simulink model "HopperPlant_optimisation"  (R2024b)
settings: Solver=VariableStepAuto  StartTime=0.0  StopTime=60  RelTol=1e-3
values from neighbouring files (symbols this model uses):
  height_setpoint = 20    [Visualisation.m]    (also in optimisation.m)
  Kd_z = 50.7347    [Visualisation.m]    (also in optimisation.m)
  Ki_z = 0.35426    [Visualisation.m]    (also in optimisation.m)
  Kp_z = 90.3674    [Visualisation.m]    (also in optimisation.m)
  max_thrust = 20    [Visualisation.m]    (also in optimisation.m)
  x_setpoint = 2    [Visualisation.m]    (also in optimisation.m)
  y_setpoint = 2    [Visualisation.m]    (also in optimisation.m)
undefined symbols (not defined in the file or in its folder): DiscIntNeverNeededParam, Kd_alpha, Kd_beta, Kd_x, Kd_y, Ki_alpha, Ki_beta, Ki_x, Ki_y, Kp_alpha, Kp_beta, Kp_x, Kp_y
libraries: slpidlib x15
(part 2 of 2)

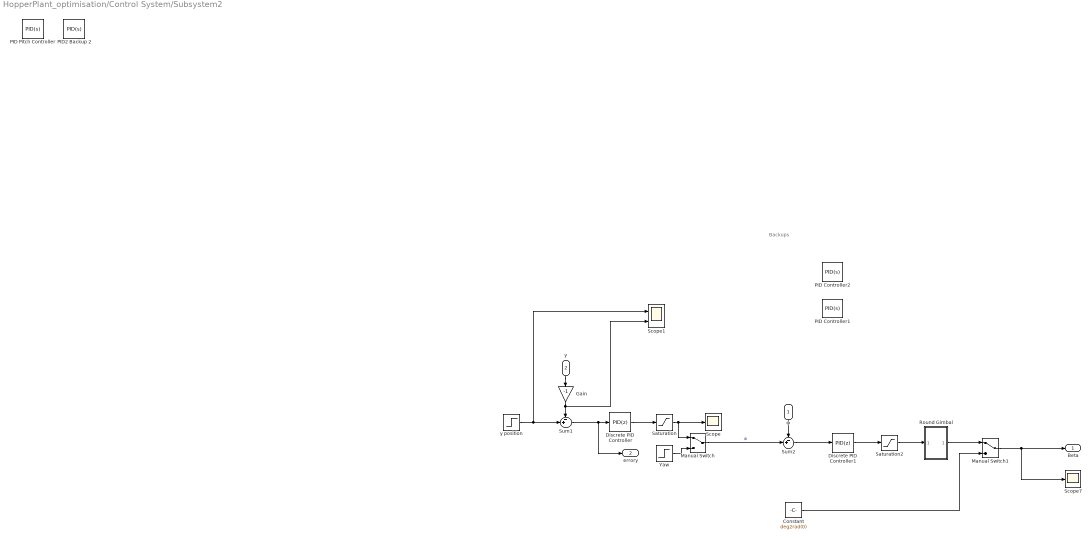
== system HopperPlant_optimisation/Control System/Subsystem2 ==
  note: Backups
  Φ : Inport
  y : Inport  Port=2
  Constant : Constant  Value=deg2rad(0)  SampleTime=0.01
  Discrete PID Controller : slpidlib/PID Controller  Controller=PID  Form=Parallel  TimeDomain=Discrete-time  UseExternalTs=off  SampleTime=-1  IntegratorMethod=Forward Euler  FilterMethod=Forward Euler  ControllerParametersSource=internal  P=Kp_y  I=Ki_y  UseKiTs=off  D=Kd_y  UseExternalDerivativeSource=off  N=100  UseFilter=off  TunerSelectOption=Transfer Function Based (PID Tuner App)  InitialConditionSource=internal  InitialConditionForIntegrator=0  InitialConditionForFilter=0  DifferentiatorICPrevScaledInput=0  ExternalReset=none  TrackingMode=off  Kt=1  LimitOutput=off  SatLimitsSource=internal  UpperSaturationLimit=inf  LowerSaturationLimit=-inf  LinearizeAsGain=off  AntiWindupMode=none  Kb=1  LimitIntegrator=off  UpperIntegratorSaturationLimit=inf  LowerIntegratorSaturationLimit=-inf  POutMin=[]  POutMax=[]  IOutMin=[]  IOutMax=[]  DOutMin=[]  DOutMax=[]  NOutMin=[]  NOutMax=[]  SumOutMin=[]  SumOutMax=[]  SaturationOutMin=[]  SaturationOutMax=[]  PParamMin=[]  PParamMax=[]  IParamMin=[]  IParamMax=[]  DParamMin=[]  DParamMax=[]  NParamMin=[]  NParamMax=[]  KbParamMin=[]  KbParamMax=[]  KtParamMin=[]  KtParamMax=[]  KbOutMin=[]  KbOutMax=[]  KtOutMin=[]  KtOutMax=[]  IntegratorOutMin=[]  IntegratorOutMax=[]  FilterOutMin=[]  FilterOutMax=[]  SumI1OutMin=[]  SumI1OutMax=[]  SumI2OutMin=[]  SumI2OutMax=[]  SumI3OutMin=[]  SumI3OutMax=[]  SumI4OutMin=[]  SumI4OutMax=[]  SumDOutMin=[]  SumDOutMax=[]  DifferentiatorOutMin=[]  DifferentiatorOutMax=[]  FilterDiffOutCoefMin=[]  FilterDiffOutCoefMax=[]  ReciprocalOutMin=[]  ReciprocalOutMax=[]  SumDenOutMin=[]  SumDenOutMax=[]  SumNumOutMin=[]  SumNumOutMax=[]  DivideOutMin=[]  DivideOutMax=[]  UdiffTsProdOutMin=[]  UdiffTsProdOutMax=[]  NTsProdOutMin=[]  NTsProdOutMax=[]  UintegralTsProdOutMin=[]  UintegralTsProdOutMax=[]  UngainTsProdOutMin=[]  UngainTsProdOutMax=[]  ClampingZeroOutDataTypeStr=Inherit: Inherit via back propagation  ClampingZeroOutMin=[]  ClampingZeroOutMax=[]  FilterDenConstantOutDataTypeStr=Inherit: Inherit via back propagation  FilterDenConstantOutMin=[]  FilterDenConstantOutMax=[]  PCopyOutDataTypeStr=Inherit: Inherit via back propagation  PCopyOutMin=[]  PCopyOutMax=[]  NCopyOutDataTypeStr=Inherit: Inherit via back propagation  NCopyOutMin=[]  NCopyOutMax=[]  IntegratorContinuousStateAttributes=''  IntegratorStateMustResolveToSignalObject=off  IntegratorRTWStateStorageClass=Auto  FilterContinuousStateAttributes=''  FilterStateMustResolveToSignalObject=off  FilterRTWStateStorageClass=Auto  ParallelPVariant=InternalParameters  IdealPVariant=Disabled  IVariant=InternalParameters  DVariant=InternalParameters  IntegratorVariant=Discrete  SatVariant=Disabled  AWVariant=Passthrough  PCopyVariant=Disabled  TRVariant=Disabled  FdbkBlocksVariant=Forward  IdealPFdbkVariant=Disabled  SatFdbkVariant=Disabled  DerivativeFilterVariant=Differentiator  NVariant=Passthrough  NCopyVariant=Disabled_SignalSpec  FilterICVariant=InternalICsDifferentiator  IntegratorICVariant=InternalICs  ExternalResetVariant=Disabled  TRSumVariant=Passthrough  SumFdbkVariant=Disabled  SumVariant=Sum_PID  TsampFilterVariant=InternalTs  TsampNgainVariant=Passthrough  TsampIntegralVariant=Disabled_SignalSpec  ExternalSaturationOutDataTypeStr=Inherit: Same as second input  DerivativeSourceVariant=ErrorSignal  PreIntVariant=InternalPreInt
      settings: LibrarySourceBlock=simulink/Discrete/Discrete PID Controller
  Discrete PID Controller1 : slpidlib/PID Controller  Controller=PID  Form=Parallel  TimeDomain=Discrete-time  UseExternalTs=off  SampleTime=-1  IntegratorMethod=Forward Euler  FilterMethod=Forward Euler  ControllerParametersSource=internal  P=Kp_beta  I=Ki_beta  UseKiTs=off  D=Kd_beta  UseExternalDerivativeSource=off  N=100  UseFilter=on  TunerSelectOption=Transfer Function Based (PID Tuner App)  InitialConditionSource=internal  InitialConditionForIntegrator=0  InitialConditionForFilter=0  DifferentiatorICPrevScaledInput=0  ExternalReset=none  TrackingMode=off  Kt=1  LimitOutput=off  SatLimitsSource=internal  UpperSaturationLimit=inf  LowerSaturationLimit=-inf  LinearizeAsGain=off  AntiWindupMode=none  Kb=1  LimitIntegrator=off  UpperIntegratorSaturationLimit=inf  LowerIntegratorSaturationLimit=-inf  POutMin=[]  POutMax=[]  IOutMin=[]  IOutMax=[]  DOutMin=[]  DOutMax=[]  NOutMin=[]  NOutMax=[]  SumOutMin=[]  SumOutMax=[]  SaturationOutMin=[]  SaturationOutMax=[]  PParamMin=[]  PParamMax=[]  IParamMin=[]  IParamMax=[]  DParamMin=[]  DParamMax=[]  NParamMin=[]  NParamMax=[]  KbParamMin=[]  KbParamMax=[]  KtParamMin=[]  KtParamMax=[]  KbOutMin=[]  KbOutMax=[]  KtOutMin=[]  KtOutMax=[]  IntegratorOutMin=[]  IntegratorOutMax=[]  FilterOutMin=[]  FilterOutMax=[]  SumI1OutMin=[]  SumI1OutMax=[]  SumI2OutMin=[]  SumI2OutMax=[]  SumI3OutMin=[]  SumI3OutMax=[]  SumI4OutMin=[]  SumI4OutMax=[]  SumDOutMin=[]  SumDOutMax=[]  DifferentiatorOutMin=[]  DifferentiatorOutMax=[]  FilterDiffOutCoefMin=[]  FilterDiffOutCoefMax=[]  ReciprocalOutMin=[]  ReciprocalOutMax=[]  SumDenOutMin=[]  SumDenOutMax=[]  SumNumOutMin=[]  SumNumOutMax=[]  DivideOutMin=[]  DivideOutMax=[]  UdiffTsProdOutMin=[]  UdiffTsProdOutMax=[]  NTsProdOutMin=[]  NTsProdOutMax=[]  UintegralTsProdOutMin=[]  UintegralTsProdOutMax=[]  UngainTsProdOutMin=[]  UngainTsProdOutMax=[]  ClampingZeroOutDataTypeStr=Inherit: Inherit via back propagation  ClampingZeroOutMin=[]  ClampingZeroOutMax=[]  FilterDenConstantOutDataTypeStr=Inherit: Inherit via back propagation  FilterDenConstantOutMin=[]  FilterDenConstantOutMax=[]  PCopyOutDataTypeStr=Inherit: Inherit via back propagation  PCopyOutMin=[]  PCopyOutMax=[]  NCopyOutDataTypeStr=Inherit: Inherit via back propagation  NCopyOutMin=[]  NCopyOutMax=[]  IntegratorContinuousStateAttributes=''  IntegratorStateMustResolveToSignalObject=off  IntegratorRTWStateStorageClass=Auto  FilterContinuousStateAttributes=''  FilterStateMustResolveToSignalObject=off  FilterRTWStateStorageClass=Auto  ParallelPVariant=InternalParameters  IdealPVariant=Disabled  IVariant=InternalParameters  DVariant=InternalParameters  IntegratorVariant=Discrete  SatVariant=Disabled  AWVariant=Passthrough  PCopyVariant=Disabled  TRVariant=Disabled  FdbkBlocksVariant=Forward  IdealPFdbkVariant=Disabled  SatFdbkVariant=Disabled  DerivativeFilterVariant=ForwardEulerFilter  NVariant=InternalParameters  NCopyVariant=Disabled  FilterICVariant=InternalICsFilter  IntegratorICVariant=InternalICs  ExternalResetVariant=Disabled  TRSumVariant=Passthrough  SumFdbkVariant=Disabled  SumVariant=Sum_PID  TsampFilterVariant=InternalTs  TsampNgainVariant=Passthrough  TsampIntegralVariant=Disabled_SignalSpec  ExternalSaturationOutDataTypeStr=Inherit: Same as second input  DerivativeSourceVariant=ErrorSignal  PreIntVariant=InternalPreInt
      settings: LibrarySourceBlock=hdlsllib/Discrete/Discrete PID Controller
  Gain : Gain  Gain=-1
  Manual Switch : ManualSwitch
  Manual Switch1 : ManualSwitch
  PID Controller1 : slpidlib/PID Controller  Controller=PID  Form=Parallel  TimeDomain=Continuous-time  UseExternalTs=off  SampleTime=-1  IntegratorMethod=Forward Euler  FilterMethod=Forward Euler  ControllerParametersSource=internal  P=0.001  I=0  UseKiTs=off  D=0.00250  UseExternalDerivativeSource=off  N=100  UseFilter=on  TunerSelectOption=Transfer Function Based (PID Tuner App)  InitialConditionSource=internal  InitialConditionForIntegrator=0  InitialConditionForFilter=0  DifferentiatorICPrevScaledInput=0  ExternalReset=none  TrackingMode=off  Kt=1  LimitOutput=off  SatLimitsSource=internal  UpperSaturationLimit=inf  LowerSaturationLimit=-inf  LinearizeAsGain=on  AntiWindupMode=none  Kb=1  LimitIntegrator=off  UpperIntegratorSaturationLimit=inf  LowerIntegratorSaturationLimit=-inf  POutMin=[]  POutMax=[]  IOutMin=[]  IOutMax=[]  DOutMin=[]  DOutMax=[]  NOutMin=[]  NOutMax=[]  SumOutMin=[]  SumOutMax=[]  SaturationOutMin=[]  SaturationOutMax=[]  PParamMin=[]  PParamMax=[]  IParamMin=[]  IParamMax=[]  DParamMin=[]  DParamMax=[]  NParamMin=[]  NParamMax=[]  KbParamMin=[]  KbParamMax=[]  KtParamMin=[]  KtParamMax=[]  KbOutMin=[]  KbOutMax=[]  KtOutMin=[]  KtOutMax=[]  IntegratorOutMin=[]  IntegratorOutMax=[]  FilterOutMin=[]  FilterOutMax=[]  SumI1OutMin=[]  SumI1OutMax=[]  SumI2OutMin=[]  SumI2OutMax=[]  SumI3OutMin=[]  SumI3OutMax=[]  SumI4OutMin=[]  SumI4OutMax=[]  SumDOutMin=[]  SumDOutMax=[]  DifferentiatorOutMin=[]  DifferentiatorOutMax=[]  FilterDiffOutCoefMin=[]  FilterDiffOutCoefMax=[]  ReciprocalOutMin=[]  ReciprocalOutMax=[]  SumDenOutMin=[]  SumDenOutMax=[]  SumNumOutMin=[]  SumNumOutMax=[]  DivideOutMin=[]  DivideOutMax=[]  UdiffTsProdOutMin=[]  UdiffTsProdOutMax=[]  NTsProdOutMin=[]  NTsProdOutMax=[]  UintegralTsProdOutMin=[]  UintegralTsProdOutMax=[]  UngainTsProdOutMin=[]  UngainTsProdOutMax=[]  ClampingZeroOutDataTypeStr=Inherit: Inherit via back propagation  ClampingZeroOutMin=[]  ClampingZeroOutMax=[]  FilterDenConstantOutDataTypeStr=Inherit: Inherit via back propagation  FilterDenConstantOutMin=[]  FilterDenConstantOutMax=[]  PCopyOutDataTypeStr=Inherit: Inherit via back propagation  PCopyOutMin=[]  PCopyOutMax=[]  NCopyOutDataTypeStr=Inherit: Inherit via back propagation  NCopyOutMin=[]  NCopyOutMax=[]  IntegratorContinuousStateAttributes=''  IntegratorStateMustResolveToSignalObject=off  IntegratorRTWStateStorageClass=Auto  FilterContinuousStateAttributes=''  FilterStateMustResolveToSignalObject=off  FilterRTWStateStorageClass=Auto  ParallelPVariant=InternalParameters  IdealPVariant=Disabled  IVariant=InternalParameters  DVariant=InternalParameters  IntegratorVariant=Continuous  SatVariant=Disabled  AWVariant=Passthrough  PCopyVariant=Disabled  TRVariant=Disabled  FdbkBlocksVariant=Forward  IdealPFdbkVariant=Disabled  SatFdbkVariant=Disabled  DerivativeFilterVariant=ContFilter  NVariant=InternalParameters  NCopyVariant=Disabled  FilterICVariant=InternalICsFilter  IntegratorICVariant=InternalICs  ExternalResetVariant=Disabled  TRSumVariant=Passthrough  SumFdbkVariant=Disabled  SumVariant=Sum_PID  TsampFilterVariant=InternalTs  TsampNgainVariant=Passthrough  TsampIntegralVariant=Disabled_SignalSpec  ExternalSaturationOutDataTypeStr=Inherit: Same as second input  DerivativeSourceVariant=ErrorSignal  PreIntVariant=InternalPreInt
  PID Controller2 : slpidlib/PID Controller  Controller=PID  Form=Parallel  TimeDomain=Continuous-time  UseExternalTs=off  SampleTime=-1  IntegratorMethod=Forward Euler  FilterMethod=Forward Euler  ControllerParametersSource=internal  P=-0.00007  I=0  UseKiTs=off  D=-0.00360  UseExternalDerivativeSource=off  N=100  UseFilter=on  TunerSelectOption=Frequency Response Based  InitialConditionSource=internal  InitialConditionForIntegrator=0  InitialConditionForFilter=0  DifferentiatorICPrevScaledInput=0  ExternalReset=none  TrackingMode=off  Kt=1  LimitOutput=off  SatLimitsSource=internal  UpperSaturationLimit=inf  LowerSaturationLimit=-inf  LinearizeAsGain=on  AntiWindupMode=none  Kb=1  LimitIntegrator=off  UpperIntegratorSaturationLimit=inf  LowerIntegratorSaturationLimit=-inf  POutMin=[]  POutMax=[]  IOutMin=[]  IOutMax=[]  DOutMin=[]  DOutMax=[]  NOutMin=[]  NOutMax=[]  SumOutMin=[]  SumOutMax=[]  SaturationOutMin=[]  SaturationOutMax=[]  PParamMin=[]  PParamMax=[]  IParamMin=[]  IParamMax=[]  DParamMin=[]  DParamMax=[]  NParamMin=[]  NParamMax=[]  KbParamMin=[]  KbParamMax=[]  KtParamMin=[]  KtParamMax=[]  KbOutMin=[]  KbOutMax=[]  KtOutMin=[]  KtOutMax=[]  IntegratorOutMin=[]  IntegratorOutMax=[]  FilterOutMin=[]  FilterOutMax=[]  SumI1OutMin=[]  SumI1OutMax=[]  SumI2OutMin=[]  SumI2OutMax=[]  SumI3OutMin=[]  SumI3OutMax=[]  SumI4OutMin=[]  SumI4OutMax=[]  SumDOutMin=[]  SumDOutMax=[]  DifferentiatorOutMin=[]  DifferentiatorOutMax=[]  FilterDiffOutCoefMin=[]  FilterDiffOutCoefMax=[]  ReciprocalOutMin=[]  ReciprocalOutMax=[]  SumDenOutMin=[]  SumDenOutMax=[]  SumNumOutMin=[]  SumNumOutMax=[]  DivideOutMin=[]  DivideOutMax=[]  UdiffTsProdOutMin=[]  UdiffTsProdOutMax=[]  NTsProdOutMin=[]  NTsProdOutMax=[]  UintegralTsProdOutMin=[]  UintegralTsProdOutMax=[]  UngainTsProdOutMin=[]  UngainTsProdOutMax=[]  ClampingZeroOutDataTypeStr=Inherit: Inherit via back propagation  ClampingZeroOutMin=[]  ClampingZeroOutMax=[]  FilterDenConstantOutDataTypeStr=Inherit: Inherit via back propagation  FilterDenConstantOutMin=[]  FilterDenConstantOutMax=[]  PCopyOutDataTypeStr=Inherit: Inherit via back propagation  PCopyOutMin=[]  PCopyOutMax=[]  NCopyOutDataTypeStr=Inherit: Inherit via back propagation  NCopyOutMin=[]  NCopyOutMax=[]  IntegratorContinuousStateAttributes=''  IntegratorStateMustResolveToSignalObject=off  IntegratorRTWStateStorageClass=Auto  FilterContinuousStateAttributes=''  FilterStateMustResolveToSignalObject=off  FilterRTWStateStorageClass=Auto  ParallelPVariant=InternalParameters  IdealPVariant=Disabled  IVariant=InternalParameters  DVariant=InternalParameters  IntegratorVariant=Continuous  SatVariant=Disabled  AWVariant=Passthrough  PCopyVariant=Disabled  TRVariant=Disabled  FdbkBlocksVariant=Forward  IdealPFdbkVariant=Disabled  SatFdbkVariant=Disabled  DerivativeFilterVariant=ContFilter  NVariant=InternalParameters  NCopyVariant=Disabled  FilterICVariant=InternalICsFilter  IntegratorICVariant=InternalICs  ExternalResetVariant=Disabled  TRSumVariant=Passthrough  SumFdbkVariant=Disabled  SumVariant=Sum_PID  TsampFilterVariant=InternalTs  TsampNgainVariant=Passthrough  TsampIntegralVariant=Disabled_SignalSpec  ExternalSaturationOutDataTypeStr=Inherit: Same as second input  DerivativeSourceVariant=ErrorSignal  PreIntVariant=InternalPreInt
  PID Pitch Controller : slpidlib/PID Controller  Controller=PID  Form=Parallel  TimeDomain=Continuous-time  UseExternalTs=off  SampleTime=-1  IntegratorMethod=Forward Euler  FilterMethod=Forward Euler  ControllerParametersSource=internal  P=-0.001  I=-0.0000011  UseKiTs=off  D=-0.015  UseExternalDerivativeSource=off  N=100  UseFilter=on  TunerSelectOption=Transfer Function Based (PID Tuner App)  InitialConditionSource=internal  InitialConditionForIntegrator=0  InitialConditionForFilter=0  DifferentiatorICPrevScaledInput=0  ExternalReset=none  TrackingMode=off  Kt=1  LimitOutput=off  SatLimitsSource=internal  UpperSaturationLimit=inf  LowerSaturationLimit=-inf  LinearizeAsGain=on  AntiWindupMode=none  Kb=1  LimitIntegrator=off  UpperIntegratorSaturationLimit=inf  LowerIntegratorSaturationLimit=-inf  POutMin=[]  POutMax=[]  IOutMin=[]  IOutMax=[]  DOutMin=[]  DOutMax=[]  NOutMin=[]  NOutMax=[]  SumOutMin=[]  SumOutMax=[]  SaturationOutMin=[]  SaturationOutMax=[]  PParamMin=[]  PParamMax=[]  IParamMin=[]  IParamMax=[]  DParamMin=[]  DParamMax=[]  NParamMin=[]  NParamMax=[]  KbParamMin=[]  KbParamMax=[]  KtParamMin=[]  KtParamMax=[]  KbOutMin=[]  KbOutMax=[]  KtOutMin=[]  KtOutMax=[]  IntegratorOutMin=[]  IntegratorOutMax=[]  FilterOutMin=[]  FilterOutMax=[]  SumI1OutMin=[]  SumI1OutMax=[]  SumI2OutMin=[]  SumI2OutMax=[]  SumI3OutMin=[]  SumI3OutMax=[]  SumI4OutMin=[]  SumI4OutMax=[]  SumDOutMin=[]  SumDOutMax=[]  DifferentiatorOutMin=[]  DifferentiatorOutMax=[]  FilterDiffOutCoefMin=[]  FilterDiffOutCoefMax=[]  ReciprocalOutMin=[]  ReciprocalOutMax=[]  SumDenOutMin=[]  SumDenOutMax=[]  SumNumOutMin=[]  SumNumOutMax=[]  DivideOutMin=[]  DivideOutMax=[]  UdiffTsProdOutMin=[]  UdiffTsProdOutMax=[]  NTsProdOutMin=[]  NTsProdOutMax=[]  UintegralTsProdOutMin=[]  UintegralTsProdOutMax=[]  UngainTsProdOutMin=[]  UngainTsProdOutMax=[]  ClampingZeroOutDataTypeStr=Inherit: Inherit via back propagation  ClampingZeroOutMin=[]  ClampingZeroOutMax=[]  FilterDenConstantOutDataTypeStr=Inherit: Inherit via back propagation  FilterDenConstantOutMin=[]  FilterDenConstantOutMax=[]  PCopyOutDataTypeStr=Inherit: Inherit via back propagation  PCopyOutMin=[]  PCopyOutMax=[]  NCopyOutDataTypeStr=Inherit: Inherit via back propagation  NCopyOutMin=[]  NCopyOutMax=[]  IntegratorContinuousStateAttributes=''  IntegratorStateMustResolveToSignalObject=off  IntegratorRTWStateStorageClass=Auto  FilterContinuousStateAttributes=''  FilterStateMustResolveToSignalObject=off  FilterRTWStateStorageClass=Auto  ParallelPVariant=InternalParameters  IdealPVariant=Disabled  IVariant=InternalParameters  DVariant=InternalParameters  IntegratorVariant=Continuous  SatVariant=Disabled  AWVariant=Passthrough  PCopyVariant=Disabled  TRVariant=Disabled  FdbkBlocksVariant=Forward  IdealPFdbkVariant=Disabled  SatFdbkVariant=Disabled  DerivativeFilterVariant=ContFilter  NVariant=InternalParameters  NCopyVariant=Disabled  FilterICVariant=InternalICsFilter  IntegratorICVariant=InternalICs  ExternalResetVariant=Disabled  TRSumVariant=Passthrough  SumFdbkVariant=Disabled  SumVariant=Sum_PID  TsampFilterVariant=InternalTs  TsampNgainVariant=Passthrough  TsampIntegralVariant=Disabled_SignalSpec  ExternalSaturationOutDataTypeStr=Inherit: Same as second input  DerivativeSourceVariant=ErrorSignal  PreIntVariant=InternalPreInt
  PID2 Backup 2 : slpidlib/PID Controller  Controller=PID  Form=Parallel  TimeDomain=Continuous-time  UseExternalTs=off  SampleTime=-1  IntegratorMethod=Forward Euler  FilterMethod=Forward Euler  ControllerParametersSource=internal  P=0.0001  I=0  UseKiTs=off  D=0.00175  UseExternalDerivativeSource=off  N=100  UseFilter=on  TunerSelectOption=Frequency Response Based  InitialConditionSource=internal  InitialConditionForIntegrator=0  InitialConditionForFilter=0  DifferentiatorICPrevScaledInput=0  ExternalReset=none  TrackingMode=off  Kt=1  LimitOutput=off  SatLimitsSource=internal  UpperSaturationLimit=inf  LowerSaturationLimit=-inf  LinearizeAsGain=on  AntiWindupMode=none  Kb=1  LimitIntegrator=off  UpperIntegratorSaturationLimit=inf  LowerIntegratorSaturationLimit=-inf  POutMin=[]  POutMax=[]  IOutMin=[]  IOutMax=[]  DOutMin=[]  DOutMax=[]  NOutMin=[]  NOutMax=[]  SumOutMin=[]  SumOutMax=[]  SaturationOutMin=[]  SaturationOutMax=[]  PParamMin=[]  PParamMax=[]  IParamMin=[]  IParamMax=[]  DParamMin=[]  DParamMax=[]  NParamMin=[]  NParamMax=[]  KbParamMin=[]  KbParamMax=[]  KtParamMin=[]  KtParamMax=[]  KbOutMin=[]  KbOutMax=[]  KtOutMin=[]  KtOutMax=[]  IntegratorOutMin=[]  IntegratorOutMax=[]  FilterOutMin=[]  FilterOutMax=[]  SumI1OutMin=[]  SumI1OutMax=[]  SumI2OutMin=[]  SumI2OutMax=[]  SumI3OutMin=[]  SumI3OutMax=[]  SumI4OutMin=[]  SumI4OutMax=[]  SumDOutMin=[]  SumDOutMax=[]  DifferentiatorOutMin=[]  DifferentiatorOutMax=[]  FilterDiffOutCoefMin=[]  FilterDiffOutCoefMax=[]  ReciprocalOutMin=[]  ReciprocalOutMax=[]  SumDenOutMin=[]  SumDenOutMax=[]  SumNumOutMin=[]  SumNumOutMax=[]  DivideOutMin=[]  DivideOutMax=[]  UdiffTsProdOutMin=[]  UdiffTsProdOutMax=[]  NTsProdOutMin=[]  NTsProdOutMax=[]  UintegralTsProdOutMin=[]  UintegralTsProdOutMax=[]  UngainTsProdOutMin=[]  UngainTsProdOutMax=[]  ClampingZeroOutDataTypeStr=Inherit: Inherit via back propagation  ClampingZeroOutMin=[]  ClampingZeroOutMax=[]  FilterDenConstantOutDataTypeStr=Inherit: Inherit via back propagation  FilterDenConstantOutMin=[]  FilterDenConstantOutMax=[]  PCopyOutDataTypeStr=Inherit: Inherit via back propagation  PCopyOutMin=[]  PCopyOutMax=[]  NCopyOutDataTypeStr=Inherit: Inherit via back propagation  NCopyOutMin=[]  NCopyOutMax=[]  IntegratorContinuousStateAttributes=''  IntegratorStateMustResolveToSignalObject=off  IntegratorRTWStateStorageClass=Auto  FilterContinuousStateAttributes=''  FilterStateMustResolveToSignalObject=off  FilterRTWStateStorageClass=Auto  ParallelPVariant=InternalParameters  IdealPVariant=Disabled  IVariant=InternalParameters  DVariant=InternalParameters  IntegratorVariant=Continuous  SatVariant=Disabled  AWVariant=Passthrough  PCopyVariant=Disabled  TRVariant=Disabled  FdbkBlocksVariant=Forward  IdealPFdbkVariant=Disabled  SatFdbkVariant=Disabled  DerivativeFilterVariant=ContFilter  NVariant=InternalParameters  NCopyVariant=Disabled  FilterICVariant=InternalICsFilter  IntegratorICVariant=InternalICs  ExternalResetVariant=Disabled  TRSumVariant=Passthrough  SumFdbkVariant=Disabled  SumVariant=Sum_PID  TsampFilterVariant=InternalTs  TsampNgainVariant=Passthrough  TsampIntegralVariant=Disabled_SignalSpec  ExternalSaturationOutDataTypeStr=Inherit: Same as second input  DerivativeSourceVariant=ErrorSignal  PreIntVariant=InternalPreInt
  Round Gimbal : Subsystem
  Saturation : Saturate  UpperLimit=deg2rad(10)  LowerLimit=-deg2rad(10)
  Saturation2 : Saturate  UpperLimit=deg2rad(10)  LowerLimit=deg2rad(-10)
  Scope : Scope
  Scope1 : Scope  NumInputPorts=2
  Scope7 : Scope
  Sum1 : Sum  Inputs=-+|
  Sum2 : Sum  Inputs=-+|
  Yaw : Step  After=0.1745  SampleTime=0
  y position : Step  Time=0  After=y_setpoint  SampleTime=0.01
  Beta : Outport
  errory : Outport  Port=2
  wires:
  Sum2/1 -> Discrete PID Controller1/1
  Discrete PID Controller1/1 -> Saturation2/1
  Φ/1 -> Sum2/1
  Saturation2/1 -> Round Gimbal/1(In1)
  y position/1 -> Scope1/1, Sum1/2
  Sum1/1 -> errory/1, Discrete PID Controller/1
  Discrete PID Controller/1 -> Saturation/1
  y/1 -> Gain/1
  Saturation/1 -> Manual Switch/1, Scope/1
  Manual Switch/1 -> Sum2/2  "Φ"
  Yaw/1 -> Manual Switch/2
  Gain/1 -> Scope1/2, Sum1/1
  Constant/1 -> Manual Switch1/2
  Manual Switch1/1 -> Scope7/1, Beta/1
  Round Gimbal/1(Out1) -> Manual Switch1/1

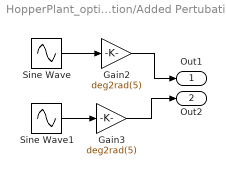
== system HopperPlant_optimisation/Pertubation/Added Pertubations ==
  Gain2 : Gain  Gain=deg2rad(5)
  Gain3 : Gain  Gain=deg2rad(5)
  Sine Wave : Sin  Frequency=0.5  SampleTime=0
  Sine Wave1 : Sin  Frequency=0.5  SampleTime=0
  Out1 : Outport
  Out2 : Outport  Port=2
  wires:
  Sine Wave1/1 -> Gain3/1
  Gain2/1 -> Out1/1
  Sine Wave/1 -> Gain2/1
  Gain3/1 -> Out2/1

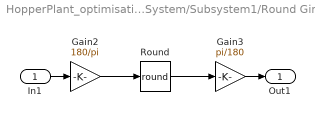
== system HopperPlant_optimisation/Control System/Subsystem1/Round Gimbal ==
  In1 : Inport
  Gain2 : Gain  Gain=180/pi
  Gain3 : Gain  Gain=pi/180
  Round : Rounding  Operator=round
  Out1 : Outport
  wires:
  Round/1 -> Gain3/1
  Gain2/1 -> Round/1
  Gain3/1 -> Out1/1
  In1/1 -> Gain2/1

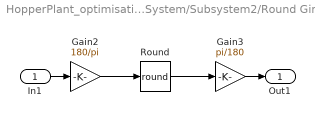
== system HopperPlant_optimisation/Control System/Subsystem2/Round Gimbal ==
  In1 : Inport
  Gain2 : Gain  Gain=180/pi
  Gain3 : Gain  Gain=pi/180
  Round : Rounding  Operator=round
  Out1 : Outport
  wires:
  Round/1 -> Gain3/1
  Gain2/1 -> Round/1
  Gain3/1 -> Out1/1
  In1/1 -> Gain2/1

== matlab function HopperPlant_optimisation/Plant/Accleration Correction ==
  data: x input; xdot input; xdot output; z input
function xdot = fcn(x,xdot, z)

phi=x(7);
theta=x(8);
psi=x(9);
T_etob=[cos(theta)*cos(psi),cos(theta)*sin(psi),-sin(theta);
    sin(theta)*sin(phi)*cos(phi)-sin(psi)*cos(phi),sin(psi)*sin(theta)*sin(phi)+cos(psi)*cos(phi), sin(phi)*cos(theta);
    sin(theta)*cos(phi)*cos(psi)+sin(psi)*sin(phi), sin(phi)*sin(theta)*cos(phi)-cos(psi)*sin(theta), cos(phi)*cos(theta)];
zddot=xdot(end);

if z <= 0 && zddot > 0
    xdot(end)=0;
    xdot(end-1)=0;
    xdot(end-2)=0;
    xdot(1:3)=T_etob*[xdot(end-2);xdot(end-1);xdot(end)];
    
end

== matlab function HopperPlant_optimisation/Plant/MATLAB Function ==
  data: x input; u input; xdot output; inertia input; cg input; thrust_pos input
function xdot   = fcn(x, u,inertia,cg, thrust_pos)
%{
Takes in thrust, angles of thrust, x and outputs xdot
Body axis is defined as z being the in the direction of gravity when pitch
is zero
mass-kg
I - moment of inertia - kg m^2
cg - centre of gravity - m
thrust position - m

x: 
U - body axis x velocity - m/s
V - body axis y velocity - m/s
W - body axis z velocity - m/s
p - body axis roll rate - rad/s
q - body axis pitch rate - rad/s
r - body axis yaw rate - rad/s
phi - earth axis roll - rad
theta - earth axis pitch - rad
psi - earth axis yaw - rad

u: 
alpha - Gimbal angle 1
beta - Gimbal angle 2
T - Thrust  

I:
dm_dt - time derivative of mass
dIxx_dt - time derivative of Ixx
dIyy_dt - time derivative of Iyy
dIzz_dt - time derivative of Izz
Ixx
Iyy
Izz
m
%}
dm_dt=inertia(1);
dIxx_dt=inertia(2);
dIyy_dt=inertia(3);
dIzz_dt=inertia(4);
Ixx=inertia(5);
Iyy=inertia(6);
Izz=inertia(7);
m=inertia(8);

%%Control input
alpha=u(1); 
beta=u(2);
T=u(3);

%%states
U=x(1);
V=x(2);
W=x(3);
p=x(4);
q=x(5);
r=x(6);
phi=x(7);
theta=x(8);
psi=x(9);


%%Constants

T_etob=[cos(theta)*cos(psi), sin(theta)*sin(phi)*cos(psi)-cos(phi)*sin(psi), cos(phi)*sin(theta)*cos(psi)+sin(phi)*sin(psi);
    cos(theta)*sin(psi), sin(phi)*sin(theta)*sin(psi)+cos(phi)*cos(psi), cos(phi)*sin(theta)*sin(psi)-sin(phi)*cos(psi);
    -sin(theta),sin(phi)*cos(theta), cos(phi)*cos(theta)]';
gb=9.81;
ge=T_etob*[0;0;gb];
gx=ge(1);
gy=ge(2);
gz=ge(3);



%%Forces

%alpha is about y and beta is about x
Tx=-T*sin(alpha);
Ty=T*cos(alpha)*sin(beta); %this should be positive,  but accounted in the gains 
Tz=-T*cos(alpha)*cos(beta);

Fx=Tx+m*gx;
Fy=Ty+m*gy;
Fz=Tz+m*gz;

%%Rotational moments
lx=thrust_pos(1)-cg(1);
ly=thrust_pos(2)-cg(2);
lz=thrust_pos(3)-cg(3);

% L=ly*Tz-lz*Ty;
% M=lx*Tz+lz*Tx;
% N=-lx*Ty-ly*Tx;

Moments=cross([lx;ly;lz],[Tx;Ty;Tz]);
L=Moments(1);
M=Moments(2);
N=Moments(3);

%%Compute xdot
Udot=Fx/m-(W*q-V*r)-dm_dt*U;
Vdot=Fy/m-(U*r-p*W)-dm_dt*V;
Wdot=Fz/m-(V*p-U*q)-dm_dt*W;

% Might Need?
% A=L+Ixz*q*p-(Izz-Iyy)*q*r;
% B=M-Ixz*(p^2-r^2)-(Ixx-Izz)*p*r;
% C=N-Ixz*q*r-(Iyy-Ixx)*p*q;
% pr_dot=[Ixx, -Ixz; -Ixz, Izz]\[A;C];
% pdot=pr_dot(1);
% qdot=B/Iyy;
% rdot=pr_dot(2);

pdot=(L-q*r*(Izz-Iyy)-dIxx_dt*p)/Ixx;
qdot=(M-r*p*(Ixx-Izz)-dIyy_dt*q)/Iyy;
rdot=(N-p*q*(Iyy-Ixx)-dIzz_dt*r)/Izz;

% Compute Euler angles
AngleCon_btoe=[1 sin(phi)*tan(theta), cos(phi)*tan(theta);
    0, cos(phi), -sin(phi); ...
    0, sin(phi)*sec(theta), cos(phi)*sec(theta)];
EulerAngledot=AngleCon_btoe*[p;q;r];

%Compute Xdot
xdot=[Udot;Vdot;Wdot;pdot;qdot; rdot;EulerAngledot];

== matlab function HopperPlant_optimisation/Inertia and Geometry/MATLAB Function1 ==
  data: delta_inertia output; dm_dt input; dm_total input; m output; mass input; geometry input; cg output; cg input
function  [delta_inertia,m,cg] = fcn(dm_dt,dm_total,mass,geometry,cg)



rho=800;
m_empty=mass(1);
m_fuel=mass(2);
R_tank=geometry(1);
A_tank=pi*R_tank^2;


C=0; %The constant from empty cg to the bottom of the fuel tank
D=0; %cg_empty * m_empty,set to 0 if axis begins at empty cg

dL_fuel=dm_total/rho*A_tank; 

L_fuel=geometry(2)-dL_fuel;


m_fuel=m_fuel+dm_total;
m=m_empty+m_fuel;

cg_fuel_z=L_fuel/2+C;
dcg_fuel_z=0.5*dL_fuel;
cg_current_z=(cg_fuel_z*m_fuel+D);
dcg_current_z=(dcg_fuel_z*m_fuel+dm_dt*cg_fuel_z/m-cg_fuel_z*m_fuel/m^2*dm_dt-D/m^2*dm_dt);
h_fuel=cg_fuel_z-cg_current_z;
dh_fuel=dcg_fuel_z-dcg_current_z;
h_empty=D/m_empty-(cg_fuel_z*m_fuel+D)/m;
dh_empty=-dcg_current_z;


cg=[cg(1),cg(2),cg_current_z];


% dIxx=1/4*dm_dt*R_tank^2+1/12*(dm_dt*L_fuel^2+2*L_fuel*dL_fuel*m_fuel)+2*h_fuel*dh_fuel*m_fuel+dm_dt*h_fuel^2+2*h_empty*dh_empty*m_empty;
dIxx=0;
dIyy=dIxx;
dx=0;
dy=0;
dIzz=1/2*dm_dt*R_tank^2+dm_dt*(dx^2+dy^2);

delta_inertia=[dm_dt,dIxx, dIyy, dIzz];

%wrong equations
% dIxx=0.25*dm_dt*R_tank^2+1/12*(dm_dt*L_fuel^2+2*L_fuel*dL_fuel*m)+2*h_fuel*dh_fuel*m+h_fuel^2*dm_dt;
% h_fuel=1/2*Lfuel-dh_fuel;
%dh_fuel=-1/2*dL_fuel;

== matlab function HopperPlant_optimisation/Plant/Velocity Correction ==
  data: x input; x output; z input; disturbance input
function x   = fcn(x, z,disturbance)

phi=x(7);
theta=x(8);
psi=x(9);
T_etob=[cos(theta)*cos(psi), sin(theta)*sin(phi)*cos(psi)-cos(phi)*sin(psi), cos(phi)*sin(theta)*cos(psi)+sin(phi)*sin(psi);
    cos(theta)*sin(psi), sin(phi)*sin(theta)*sin(psi)+cos(phi)*cos(psi), cos(phi)*sin(theta)*sin(psi)-sin(phi)*cos(psi);
    -sin(theta),sin(phi)*cos(theta), cos(phi)*cos(theta)]';


velocity=T_etob\[x(1);x(2);x(3)];
% velocity=velocity+delta;
% x(7)=x(7)+disturbance(1);
% x(8)=x(8)+disturbance(2);
if z <= 0 && velocity(3) > 0
    velocity=[0;0;0];
    x(4)=0;
    x(5)=0;
    x(6)=0;
    x(7)=x(7);
    x(8)=x(8);
    x(9)=x(9);
    x(1:3)=T_etob*velocity;
   
end

== matlab function HopperPlant_optimisation/Inertia and Geometry/Update Inertia ==
  data: delta_inertia_instant input; inertia output; delta_inertia_total input; m input; I input
function inertia  = fcn(delta_inertia_instant,delta_inertia_total,m,I)

%%Mass and inertia



Ixx=I(1);
Iyy=I(2);
Izz=I(3);


%compute change in mass and inertia using parallel axis theorems



%update Ixx, Iyy and Izz 
Ixx=Ixx+delta_inertia_total(1);
Iyy=Iyy+delta_inertia_total(2);
Izz=Izz+delta_inertia_total(3);

inertia=[delta_inertia_instant,Ixx Iyy, Izz,m];

== matlab function HopperPlant_optimisation/Plant/Convert to body axis ==
  data: velocity output; x input
function velocity = fcn(x)

phi=x(7);
theta=x(8);
psi=x(9);
T_etob=[cos(theta)*cos(psi), sin(theta)*sin(phi)*cos(psi)-cos(phi)*sin(psi), cos(phi)*sin(theta)*cos(psi)+sin(phi)*sin(psi);
    cos(theta)*sin(psi), sin(phi)*sin(theta)*sin(psi)+cos(phi)*cos(psi), cos(phi)*sin(theta)*sin(psi)-sin(phi)*cos(psi);
    -sin(theta),sin(phi)*cos(theta), cos(phi)*cos(theta)]';

velocity=T_etob\[x(1);x(2);x(3)];

== matlab function HopperPlant_optimisation/Inertia and Geometry/MATLAB Function ==
  data: mass output; geometry output; cg output; thrust_pos output; I output
function [mass, geometry,cg,thrust_pos,I] = fcn()


% % mass for hopper
% m_fuel=0;
% m_empty=40;
% % R_tank=units(152.4/2,'mm','m');
% % L_fuel=units(489,'mm','m')
% 
% R_tank=units(0,'mm','m');
% L_fuel=units(0,'mm','m');
% 
% Ixx=units(0.296,'mm^4','m^4');
% Iyy=units(0.278,'mm^4','m^4');
% Izz=units(0.1,'mm^4','m^4');
% 
% cg=[0,0,units(0,'mm','m')];
% thrust_pos=[units(0,'mm','m'),units(0,'mm','m'),units(550,'mm','m')];
% 
% mass=[m_fuel,m_empty];
% geometry=[R_tank,L_fuel];
% I=[Ixx,Iyy,Izz];

%mass property for demonstator
m_fuel=0;
m_empty=1.4;
% R_tank=units(152.4/2,'mm','m');
% L_fuel=units(489,'mm','m')

R_tank=units(0,'mm','m');
L_fuel=units(0,'mm','m');

Ixx=units(0.296,'m^4','m^4');
Iyy=units(0.296,'m^4','m^4');
Izz=units(0.05,'m^4','m^4');

cg=[0,0,units(0,'mm','m')];
thrust_pos=[units(0,'mm','m'),units(0,'mm','m'),units(72,'mm','m')];

mass=[m_fuel,m_empty];
geometry=[R_tank,L_fuel];
I=[Ixx,Iyy,Izz];
